simulink model "readDataiWalker"  (R2014a)
settings: Solver=ode45  StartTime=0.0  StopTime=Inf  RelTol=1e-3
InitFcn:
  | Ts = 0.01;
  | lid = LIDAR();
  | rob = DifferentialRobot();
  | rob.dt = 0.01;
  | rob.attachLidar(lid, [0.6,0,0]);
  | 
  | map = LandmarkMap('test');
  | V = diag([0.005, 0.1*pi/180].^2);
  | P0 = diag([0.05, 0.05, 0.01].^2);
  | W = diag([0.05, 3*pi/180].^2);
  | ekf = EKFSLAM(rob, V, P0, 'map', map, 'estMap', true, 'W', W);
  | 
  | gh = figure;
  | axis equal;
  | hold on;
  | whitebg([0 0 0]);
  | grid on;
  | 
  | pl = Plotter(gh);
undefined symbols (not defined in the file): stepWheelsUpdate
libraries: iWalkerLib x2
settings Model: Creator=Brian  LastModifiedBy=Brian

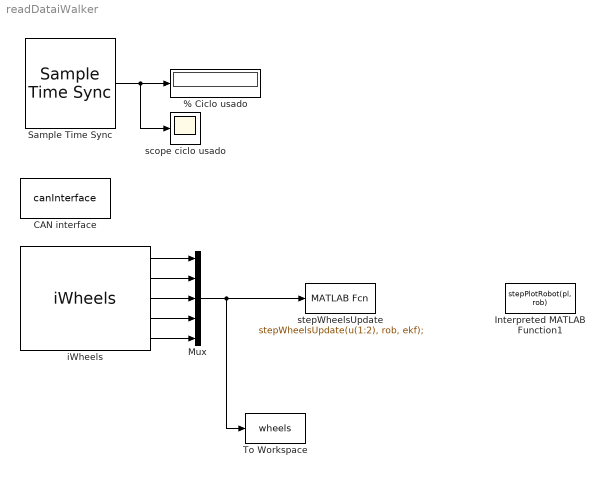
== system readDataiWalker ==
  % Ciclo usado : Display
      settings: Decimation=100
  CAN interface : S-Function  FunctionName=canInterface  EnableBusSupport=off
  Interpreted MATLAB Function1 : MATLABFcn  MATLABFcn=stepPlotRobot(pl, rob)  OutputDimensions=0  SampleTime=1/24
  Mux : Mux  Inputs=5
  Sample Time Sync : iWalkerLib/Sample Time Sync  Priority=8
  To Workspace : ToWorkspace  VariableName=wheels  SaveFormat=Timeseries  SampleTime=-1
  iWheels : iWalkerLib/iWheels  SampleTime=0.01
  scope ciclo usado : Scope
      settings: TimeRange=0.7489177489177488  YMin=0  YMax=250
  stepWheelsUpdate : MATLABFcn  MATLABFcn=stepWheelsUpdate(u(1:2), rob, ekf);  OutputDimensions=0
  wires:
  Sample Time Sync/1 -> scope ciclo usado/1, % Ciclo usado/1
  Mux/1 -> To Workspace/1, stepWheelsUpdate/1
  iWheels/2 -> Mux/2
  iWheels/3 -> Mux/3
  iWheels/4 -> Mux/4
  iWheels/5 -> Mux/5
  iWheels/1 -> Mux/1
